simulink model "EnableMotors"  (R2019b)
settings: Solver=VariableStepAuto  StartTime=0.0  StopTime=10.0  RelTol=1e-3
settings Model: Creator=Duin home  LastModifiedBy=Duin home

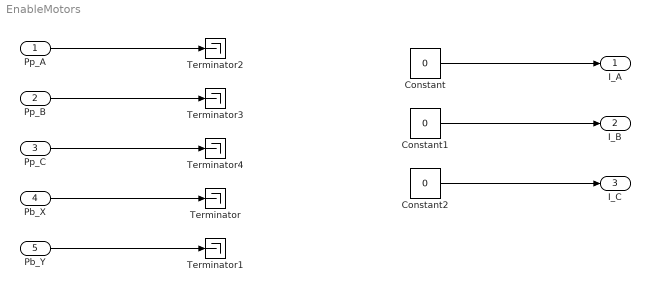
== system EnableMotors ==
  Pp_A : Inport
  Pp_B : Inport  Port=2
  Pp_C : Inport  Port=3
  Pb_X : Inport  Port=4
  Pb_Y : Inport  Port=5
  Constant : Constant  Value=0
  Constant1 : Constant  Value=0
  Constant2 : Constant  Value=0
  Terminator{,1..4} (5 alike) : Terminator
  I_A : Outport
  I_B : Outport  Port=2
  I_C : Outport  Port=3
  wires:
  Pp_C/1 -> Terminator4/1
  Pp_B/1 -> Terminator3/1
  Constant2/1 -> I_C/1
  Constant1/1 -> I_B/1
  Pb_Y/1 -> Terminator1/1
  Pp_A/1 -> Terminator2/1
  Pb_X/1 -> Terminator/1
  Constant/1 -> I_A/1
